simulink model "aula1_R2018"  (R2018a)
settings: Solver=FixedStepAuto  StartTime=0.0  StopTime=0.8  RelTol=1e-3
values from neighbouring files (symbols this model uses):
  wn = 10    [aula1_teste.m]
settings Model: Creator=celsojosemunaro  LastModifiedBy=celsojosemunaro
settings DataIOCC: ReturnWorkspaceOutputs=on
settings SFSimCC: SimUseLocalCustomCode=on
settings RTWCC: RTWUseLocalCustomCode=on

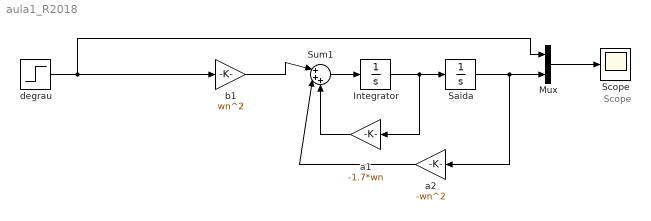
== system aula1_R2018 ==
  note: Scope
  Integrator : Integrator
  Mux : Mux  Inputs=2
  Saida : Integrator
  Scope : Scope
  Sum1 : Sum  Inputs=|+++
  a1 : Gain  Gain=-1.7*wn
  a2 : Gain  Gain=-wn^2
  b1 : Gain  Gain=wn^2
  degrau : Step  Time=0  SampleTime=0
  wires:
  Mux/1 -> Scope/1
  degrau/1 -> b1/1, Mux/1
  Sum1/1 -> Integrator/1
  Integrator/1 -> a1/1, Saida/1
  Saida/1 -> a2/1, Mux/2
  a1/1 -> Sum1/3
  a2/1 -> Sum1/2
  b1/1 -> Sum1/1
